simulink model "ACTimeOvercurrentRelayBlock_org"  (Simulink 10.0)
settings: Solver=ode23tb  StartTime=0.0  StopTime=1  RelTol=1e-3  EnableMultiTasking=on
libraries: powerlib x8, powerlib_meascontrol x1
settings Model: Creator=Rodney Tan  LastModifiedBy=bhisma
settings DataIOCC: LimitDataPoints=on
settings DebuggingCC: UnderspecifiedInitializationDetection=Simplified  MergeDetectMultiDrivingBlocksExec=error
settings GRTTargetCC: GeneratePreprocessorConditionals=Disable all  CombineOutputUpdateFcns=on  GRTInterface=off
settings ConfigComp: CovExternalEMLEnable=off
settings SimscapeCC: SimscapeNormalizeSystem=off

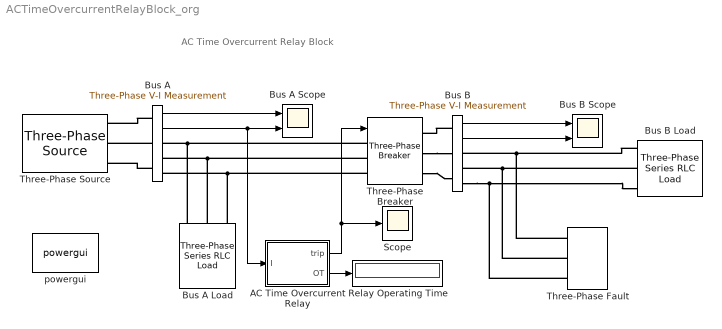
== system ACTimeOvercurrentRelayBlock_org ==
  note: AC Time Overcurrent Relay Block
  AC Time Overcurrent Relay : Subsystem  mask(AC Time Overcurrent Relay Block){tcpopup=IEC Standard Inverse, k=0.14, alpha=0.02, B=0, PS=100%, TMS=0.1, TDS=0.1, CTpri=300, CTsec=5, Freq=50, RMSInit=0}
      mask prompts: tcpopup "Trip Characteristic"; PS "Plug Setting (PS) / Low-set (I >)"; TMS "Time Multiplier Setting (TMS)"; TDS "Time Delay Setting (TDS) in sec"; CTpri "Current Transformer Primary (A)"; CTsec "Current Transformer Secondary (A)"; Freq "Fundamental frequency (Hz):"; RMSInit "Initial RMS value:"
      mask help:
      | AC Time Overcurrent Relay Block developed by Dr Rodney Tan
      | Version 1.0 (Jun 2016)
      |
      | AC Time Overcurrent Relay (ANSI/IEEE C37.2 device number 51) that operates when the current exceeds a predetermined value.
      |
      | This relay operates with either a Definite Minimum Time (DMT) or Inverse Definite Minimum Time (IDMT) characteristic.
      |
      | This relay support both IEC 60255 Standard and IEEE Standard C37.112-1996 IDMT trip characteristic.
      mask Help:
      | <b><u>Block Setting</u></b>
      | <b>Trip Characteristic</b>
      | Relay operation mode selection of Definite Minimum Time (DMT), IEC 60255 Standard or IEEE Standard C37.112-1996 Inverse Definite Minimum Time (IDMT).
      | 
      | <b>Plug-Setting(PS) / Low-set (I >)</b>
      | Specify relay pick-up current based on current transformer rating ranging from 25% to 200% with 25% step interval.
      | 
      | <b>Time Multiplier Setting (TMS)</b>
      | Specify time delay multiplier ranging from 0.05 to 1.0 for IDMT relay operation. This setting will be disabled DMT relay operation mode.
      | 
      | <b>Plot Curve Button</b>
      | Plot current Inverse Definite Minimum Time trip curve.
      | 
      | <b>Time Delay Setting (TDS)</b>
      | Specify time delay ranging from 0.05sec to 99sec for Definite Minimum Time relay operation. This setting will be disabled in IDMT relay operation mode.
      | 
      | <b>Current Transformer Primary (A)</b>
      | Specify current transformer primary in Ampere.
      | 
      | <b>Current Transformer Secondary (A)</b>
      | Specify current transformer secondary in Ampere.
      | 
      | <b>Fundamental Frequency (Hz)</b>
      | Specify the RMS current measurement fundamental frequency, in hertz, of the input signal.
      | 
      | <b>Initial RMS Value</b>
      | Specify the RMS current measurement initial RMS value of the output signal.
      | 
      | <b><u>Block Input Output</u></b>
      | <b>I</b>
      | Current input to the AC time overcurrent relay
      | 
      | <b>trip</b>
      | Trip control signal output (1-0), commonly connected to circuit breaker
      | 
      | <b>OT</b>
      | Relay operating time output
      mask TypeOptions tcpopup: Definite Minimum Time | IEC Standard Inverse | IEC Very Inverse | IEC Long Time Inverse | IEC Extremely Inverse | IEC Ultra Inverse | IEEE Moderately Inverse | IEEE Very Inverse | IEEE Extremely Inverse
      mask Callback tcpopup:
      | switch(get_param(gcb,'tcpopup'))
      |     case 'IEC Standard Inverse'
      |         set_param(gcb,'k','0.14');
      |         set_param(gcb,'alpha','0.02');
      |         set_param(gcb,'B','0');
      |         set_param(gcb,'MaskEnables',{'on','off','off','off',...
      |                   'on','on','off','on','on','on','on'});
      |     case 'IEC Very Inverse'
      |         set_param(gcb,'k','13.5');
      |         set_param(gcb,'alpha','1');
      |         set_param(gcb,'B','0');
      |         set_param(gcb,'MaskEnables',{'on','off','off','off',...
      |                   'on','on','off','on','on','on','on'});
      |     case 'IEC Long Time Inverse'
      |         set_param(gcb,'k','120');
      |         set_param(gcb,'alpha','1');
      |         set_param(gcb,'B','0');
      |         set_param(gcb,'MaskEnables',{'on','off','off','off',...
      |                   'on','on','off','on','on','on','on'});
      |     case 'IEC Extremely Inverse'
      |         set_param(gcb,'k','80');
      |         set_param(gcb,'alpha','2');
      |         set_param(gcb,'B','0');
      |         set_param(gcb,'MaskEnables',{'on','off','off','off',...
      |                   'on','on','off','on','on','on','on'});
      |     case 'IEC Ultra Inverse'
      |         set_param(gcb,'k','315.2');
      |         set_param(gcb,'alpha','2.5');
      |         set_param(gcb,'B','0');
      |         set_param(gcb,'MaskEnables',{'on','off','off','off',...
      |                   'on','on','off','on','on','on','on'});
      |     case 'IEEE Moderately Inverse'
      |         set_param(gcb,'k','0.0515');
      |         set_param(gcb,'alpha','0.02');
      |         set_param(gcb,'B','0.114');
      |         set_param(gcb,'MaskEnables',{'on','off','off','off',...
      |                   'on','on','off','on','on','on','on'});
      |     case 'IEEE Very Inverse'
      |         set_param(gcb,'k','19.61');
      |         set_param(gcb,'alpha','2');
      |         set_param(gcb,'B','0.491');
      |         set_param(gcb,'MaskEnables',{'on','off','off','off',...
      |                   'on','on','off','on','on','on','on'});
      |     case 'IEEE Extremely Inverse'
      |         set_param(gcb,'k','28.2');
      |         set_param(gcb,'alpha','2');
      |         set_param(gcb,'B','0.1217');
      |         set_param(gcb,'MaskEnables',{'on','off','off','off',...
      |                   'on','on','off','on','on','on','on'});
      |     otherwise
      |         set_param(gcb,'k','0');
      |         set_param(gcb,'MaskEnables',{'on','off','off','off',...
      |                   'on','off','on','on','on','on','on'});
      | end
      mask TypeOptions PS: 25% | 50% | 75% | 100% | 125% | 150% | 175% | 200%
      mask TypeOptions TMS: 0.05 | 0.1 | 0.15 | 0.2 | 0.25 | 0.3 | 0.35 | 0.4 | 0.45 | 0.5 | 0.55 | 0.6 | 0.65 | 0.7 | 0.75 | 0.8 | 0.85 | 0.9 | 0.95 | 1.0
      mask Callback TDS:
      | TDS = str2double(get_param(gcb,'TDS'));
      | if (TDS > 99)||(TDS < 0.05)||isnan(TDS)
      |     msgbox('TDS must be in the range of 0.05-99 sec',...
      |     'Invalid Value !','error');
      |     set_param(gcb,'TDS','0.1');
      | end
      mask TypeOptions Freq: Irms/Freq
      mask TypeOptions RMSInit: Irms/RMSInit
      mask DialogControl plotbutton Prompt: Plot Curve
      mask DialogControl plotbutton Callback:
      | % Plotting IDMT Curve
      | TMS = str2num(get_param(gcb,'TMS'));
      | k = str2num(get_param(gcb,'k'));
      | alpha = str2num(get_param(gcb,'alpha'));
      | B = str2num(get_param(gcb,'B'));
      | I = 1:20;
      | td = ((k./((I.^alpha)-1))+B)*TMS;
      | loglog(td);
      | set(gcf, 'Position', [200 150 300 500]);
      | switch(get_param(gcb,'tcpopup'))
      |     case 'IEC Standard Inverse'
      |         title('IEC Standard Inverse');
      |         set(gca, 'YTick', (1:10));
      |         ylim([0.1 10]);
      |     case 'IEC Very Inverse'
      |         title('IEC Very Inverse');
      |         set(gca, 'YTick', (1:2:15));
      |         ylim([0.01 15]);
      |     case 'IEC Long Time Inverse'
      |         title('IEC Long Time Inverse');
      |         set(gca, 'YTick', (0:20:120));
      |         ylim([0.1 120]);
      |     case 'IEC Extremely Inverse'
      |         title('IEC Extremely Inverse');
      |         set(gca, 'YTick', (0:5:30));
      |         ylim([0.01 30]);
      |     case 'IEC Ultra Inverse'
      |         title('IEC Ultra Inverse');
      |         set(gca, 'YTick', (0:20:100));
      |         ylim([0.01 100]);
      |     case 'IEEE Moderately Inverse'
      |         title('IEEE Moderately Inverse');
      |         set(gca, 'YTick', (1:5));
      |         ylim([0.01 5]);
      |     case 'IEEE Very Inverse'
      |         title('IEEE Very Inverse');
      |         set(gca, 'YTick', (1:10));
      |         ylim([0.01 10]);
      |     case 'IEEE Extremely Inverse'
      |         title('IEEE Extremely Inverse');
      |         set(gca, 'YTick', (1:10));
      |         ylim([0.01 10]);
      | end
      | 
      | set(gca, 'XTick', [1:10 20]);
      | xlim([1 30]);
      | xlabel('Current (Multiples of Plug Setting)');
      | ylabel('Operating Time (sec)');
      | grid on;
      mask DialogControl RMS Prompt: RMS Current Measurement
      mask Display:
      | disp('(51)');
      | port_label('input', 1, 'I');
      | port_label('output', 1, 'trip');
      | port_label('output', 2, 'OT');
  Bus A : powerlib/Measurements/Three-Phase V-I Measurement  VoltageMeasurement=phase-to-ground  SetLabelV=off  LabelV=Vabc  Vpu=off  VpuLL=off  CurrentMeasurement=yes  SetLabelI=off  LabelI=Iabc  Ipu=off  Pbase=100e6  Vbase=500e3  OutputType=Complex  PhasorSimulation=off  PSBequivalent=0
      settings: SourceProductName=Simscape Electrical
  Bus A Load : powerlib/Elements/Three-Phase Series RLC Load  LConnTagsString=A|B|C  Configuration=Y (grounded)  NominalVoltage=400  Vabc=[1e3 1e3 1e3]  Vabcp=[1e3 1e3 1e3]  NominalFrequency=50  UnbalancedPower=off  ActivePower=100e3  InductivePower=1000  CapacitivePower=0  Pabc=[10e3 9e3 11e3]  QLabc=[100 90 110]  QCabc=[100 90 110]  Pabcp=[10e3 9e3 11e3]  QLabcp=[100 90 110]  QCabcp=[100 90 110]  Measurements=None  LoadType=constant Z
      settings: SourceProductName=Simscape Electrical
  Bus A Scope : Scope  NumInputPorts=2
  Bus B : powerlib/Measurements/Three-Phase V-I Measurement  VoltageMeasurement=phase-to-ground  SetLabelV=off  LabelV=Vabc  Vpu=off  VpuLL=off  CurrentMeasurement=yes  SetLabelI=off  LabelI=Iabc  Ipu=off  Pbase=100e6  Vbase=500e3  OutputType=Complex  PhasorSimulation=off  PSBequivalent=0
      settings: SourceProductName=Simscape Electrical
  Bus B Load : powerlib/Elements/Three-Phase Series RLC Load  LConnTagsString=A|B|C  Configuration=Y (grounded)  NominalVoltage=400  Vabc=[1e3 1e3 1e3]  Vabcp=[1e3 1e3 1e3]  NominalFrequency=50  UnbalancedPower=off  ActivePower=100e3  InductivePower=1000  CapacitivePower=0  Pabc=[10e3 9e3 11e3]  QLabc=[100 90 110]  QCabc=[100 90 110]  Pabcp=[10e3 9e3 11e3]  QLabcp=[100 90 110]  QCabcp=[100 90 110]  Measurements=None  LoadType=constant Z
      settings: SourceProductName=Simscape Electrical
  Bus B Scope : Scope  NumInputPorts=2
  Relay Operating Time : Display
  Scope : Scope
  Three-Phase Breaker : powerlib/Elements/Three-Phase Breaker  InitialState=closed  SwitchA=on  SwitchB=on  SwitchC=on  SwitchTimes="[1/60  5/60]"  External=on  BreakerResistance=0.01  SnubberResistance=1e6  SnubberCapacitance=inf  Measurements=None
      settings: SourceProductName=Simscape Electrical
  Three-Phase Fault : powerlib/Elements/Three-Phase Fault  InitialStates=0  FaultA=on  FaultB=on  FaultC=on  GroundFault=on  SwitchTimes=0.1  External=off  SwitchStatus=NaN  FaultResistance=0.001  GroundResistance=0.01  SnubberResistance=1e6  SnubberCapacitance=inf  Measurements=None
      settings: SourceProductName=Simscape Electrical
  Three-Phase Source : powerlib/Electrical Sources/Three-Phase Source  InternalConnection=Yg  VoltagePhases=off  Voltage=400  PhaseAngle=0  Voltage_phases=[25e3 25e3 25e3]/sqrt(3)  PhaseAngles_phases=[0 -120 +120]  Frequency=50  NonIdealSource=on  SpecifyImpedance=on  Resistance=0.8929  Inductance=16.58e-3  ShortCircuitLevel=1e6  BaseVoltage=400  XRratio=7  BusType=swing  Pref=0  Qref=0  Prefabc=[10e3, 10e3, 10e3]  Qrefabc=[0, 0, 0]  Qmin=-inf  Qmax=inf
      settings: SourceProductName=Simscape Electrical
  powergui : powerlib/powergui  Priority=1  SimulationMode=Continuous  SampleTime=50e-6  frequency=60  Iterations=50  frequencyindice=50  Pbase=100e6  ErrMax=1e-4  UnitsV=kV  UnitsW=MW  buscounter=0  FunctionMessages=off  echomessages=off  EnableUseOfTLC=off  CurrentSourceSwitches=off  DisableSnubberDevices=on  DisableRonSwitches=off  DisableVfSwitches=off  DisplayEquations=off  AutomaticDiscreteSolvers=off  SolverType=Tustin/Backward Euler (TBE)  Interpol=off  ExternalGateDelay=off  methode=off  Ts=100  x0status=blocks  SPID=on  SwTol=0  HookPort=off  NonlinearTolerance=1e-4  nMaxIteration=100  ContinueOnMaxIteration=off  RestoreLinks=warning  ResistiveCurrentMeasurement=off  Frange=[0:2:500]  Ylog=off  Xlog=on  ShowGrid=off  save=off  variable=ZData  structure=0  ZoomFFT=off  StartTime=0.0  cycles=1  DisplayStyle=1  fundamental=60  FreqAxis=off  MaxFrequency=1000  frequencyindicesteady=1  RmsSteady=1  display=off
      settings: SourceProductName=Simscape Electrical
  wires:
  Bus A/2 -> Bus A Scope/2, AC Time Overcurrent Relay/1(I)
  AC Time Overcurrent Relay/1(trip) -> Three-Phase Breaker/1, Scope/1
  Bus A/1 -> Bus A Scope/1
  Bus B/1 -> Bus B Scope/1
  Bus B/2 -> Bus B Scope/2
  AC Time Overcurrent Relay/2(OT) -> Relay Operating Time/1
  connections:
  Bus A/LConn1 -- Three-Phase Source/RConn1
  Three-Phase Breaker/LConn2 -- Bus A Load/LConn2 -- Bus A/RConn2
  Three-Phase Breaker/LConn1 -- Bus A Load/LConn1 -- Bus A/RConn1
  Bus A/LConn2 -- Three-Phase Source/RConn2
  Bus A/LConn3 -- Three-Phase Source/RConn3
  Three-Phase Breaker/LConn3 -- Bus A Load/LConn3 -- Bus A/RConn3
  Three-Phase Breaker/RConn2 -- Bus B/LConn2
  Bus B/LConn1 -- Three-Phase Breaker/RConn1
  Three-Phase Breaker/RConn3 -- Bus B/LConn3
  Bus B Load/LConn2 -- Three-Phase Fault/LConn2 -- Bus B/RConn2
  Bus B/RConn3 -- Bus B Load/LConn3 -- Three-Phase Fault/LConn3
  Bus B Load/LConn1 -- Three-Phase Fault/LConn1 -- Bus B/RConn1

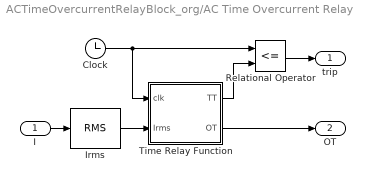
== system ACTimeOvercurrentRelayBlock_org/AC Time Overcurrent Relay ==
  I : Inport
  Clock : Clock
  Irms : powerlib_meascontrol/Measurements/RMS  TrueRMS=on  Freq=Freq  RMSInit=RMSInit  Ts=0
      settings: SourceProductName=Simscape Electrical
  Relational Operator : RelationalOperator  Operator=<=  OutDataTypeStr=boolean  RndMeth=Nearest
  Time Relay Function : MATLAB Function  TreatAsAtomicUnit=on
  trip : Outport
  OT : Outport  Port=2
  wires:
  Clock/1 -> Relational Operator/1, Time Relay Function/1(clk)
  Irms/1 -> Time Relay Function/2(Irms)
  Time Relay Function/1(TT) -> Relational Operator/2
  Time Relay Function/2(OT) -> OT/1
  Relational Operator/1 -> trip/1
  I/1 -> Irms/1

== matlab function AC Time Overcurrent Relay/Time Relay Function ==
  data: TT output double; clk input double; Irms input double; CTpri parameter double; CTsec parameter double; PS parameter double; OT output double; TMS parameter double; k parameter double; alpha parameter double; B parameter double; TDS parameter double
function [TT, OT] = fcn(clk,Irms,CTpri,CTsec,PS,TMS,k,alpha,B,TDS)

persistent RelayState TripTime OperatingTime PickupTime

if isempty(RelayState)
    RelayState = 0;
    TripTime = inf;
    OperatingTime = inf;
    PickupTime = 0;
end

CT = max(Irms/(CTpri/CTsec));
Pickup = (PS*0.25)*CTsec;

if (RelayState == 0)&&(CT > Pickup)
    PickupTime = clk;
    RelayState = 1;
end

if (RelayState == 1)&&(clk>(PickupTime+0.02)) % Wait for 20ms fault current rise time
    if k == 0
        OperatingTime = TDS;
    else
        PMS = CT/Pickup;                          % Calculate Plug Multiplier Setting
        OperatingTime = ((k/((PMS^alpha)-1))+B)*(TMS*0.05); % Determine Definite Inverse Minimum Time
    end
    TripTime = PickupTime + OperatingTime;
    RelayState = 2;
end

TT = TripTime;
OT = OperatingTime;
